simulink model "DIIFERENTATIAL_EQA"  (R2020b)
settings: Solver=FixedStepAuto  StartTime=0.0  StopTime=10.0  RelTol=1e-3
undefined symbols (not defined in the file): B, J, K, L, R
settings Model: Creator=99003740  LastModifiedBy=99003740

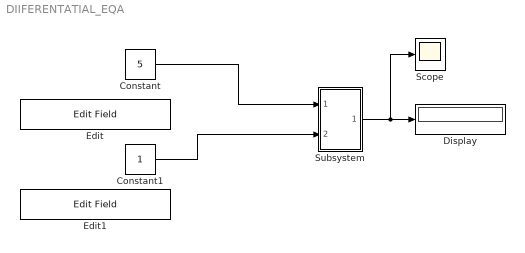
== system DIIFERENTATIAL_EQA ==
  Constant : Constant  Value=5
  Constant1 : Constant
  Display : Display
  Edit : EditField  LabelPosition=Hide  ShowInitialText=on  Alignment=Center
  Edit1 : EditField  LabelPosition=Hide  ShowInitialText=on  Alignment=Center
  Scope : Scope
  Subsystem : Subsystem
  wires:
  Constant/1 -> Subsystem/1(In1)
  Constant1/1 -> Subsystem/2(In2)
  Subsystem/1(Out1) -> Scope/1, Display/1

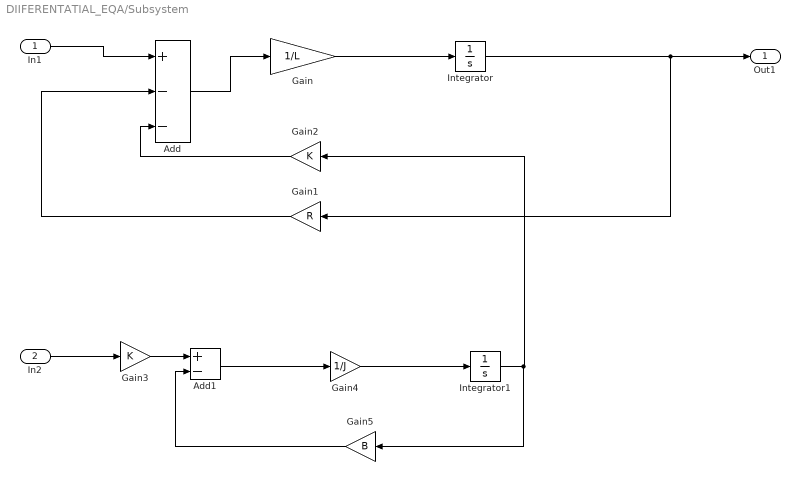
== system DIIFERENTATIAL_EQA/Subsystem ==
  In1 : Inport
  In2 : Inport  Port=2
  Add : Sum  Inputs=+--
  Add1 : Sum  Inputs=+-
  Gain : Gain  Gain=1/L
  Gain1 : Gain  Gain=R
  Gain2 : Gain  Gain=K
  Gain3 : Gain  Gain=K
  Gain4 : Gain  Gain=1/J
  Gain5 : Gain  Gain=B
  Integrator : Integrator
  Integrator1 : Integrator
  Out1 : Outport
  wires:
  Add1/1 -> Gain4/1
  Integrator/1 -> Out1/1, Gain1/1
  Gain1/1 -> Add/2
  Integrator1/1 -> Gain5/1, Gain2/1
  Gain3/1 -> Add1/1
  Gain/1 -> Integrator/1
  Gain4/1 -> Integrator1/1
  In2/1 -> Gain3/1
  Gain5/1 -> Add1/2
  Add/1 -> Gain/1
  Gain2/1 -> Add/3
  In1/1 -> Add/1
